simulink model "decoder_microinstruction_counter"  (R2020a)
settings: Solver=VariableStepAuto  StartTime=0.0  StopTime=inf  RelTol=1e-3
libraries: simulink_extras x1, dspswit3 x1, commutil2 x1
settings Model: EnablePacing=on  PacingRate=0.900000  Creator=F1  LastModifiedBy=F1

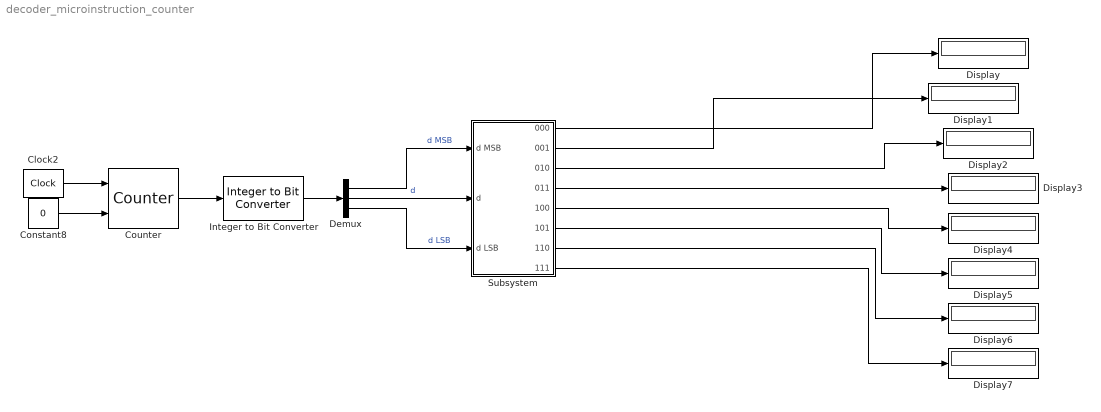
== system decoder_microinstruction_counter ==
  Clock2 : simulink_extras/Flip Flops/Clock  period=2
  Constant8 : Constant  Value=0
  Counter : dspswit3/Counter  Direction=Up  CountEvent=Rising edge  CounterSize=User defined  MaxCount=6  InitialCount=0  Output=Count  HitValue=32  ResetInput=on  SamplesPerFrame=1  Ts=1  CntDtype=int16  HitDtype=Logical
  Demux : Demux  Outputs=3
  Display{,1..7} (8 alike) : Display
  Integer to Bit Converter : commutil2/Integer to Bit Converter  nbits=3  signedInputValues=Unsigned  bitOrder=MSB first  outDtype=Inherit via internal rule
  Subsystem : Subsystem
  wires:
  Clock2/1 -> Counter/1
  Counter/1 -> Integer to Bit Converter/1
  Integer to Bit Converter/1 -> Demux/1
  Constant8/1 -> Counter/2
  Demux/1 -> Subsystem/1(d MSB)  "d MSB"
  Demux/2 -> Subsystem/2(d)  "d"
  Demux/3 -> Subsystem/3(d LSB)  "d LSB"
  Subsystem/1(000) -> Display/1
  Subsystem/2(001) -> Display1/1
  Subsystem/3(010) -> Display2/1
  Subsystem/4(011) -> Display3/1
  Subsystem/5(100) -> Display4/1
  Subsystem/6(101) -> Display5/1
  Subsystem/7(110) -> Display6/1
  Subsystem/8(111) -> Display7/1

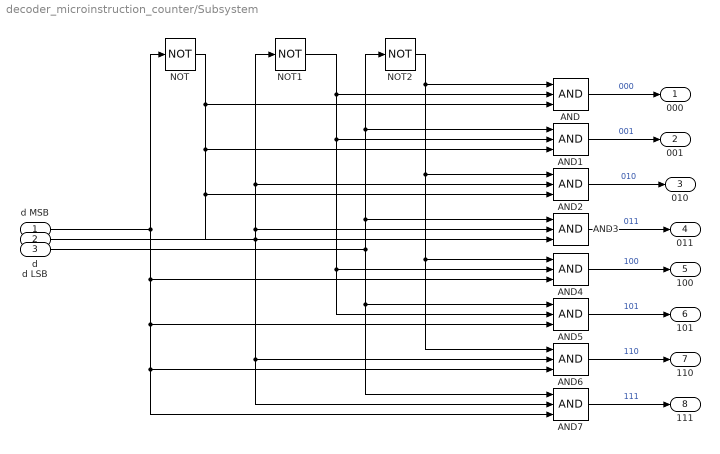
== system decoder_microinstruction_counter/Subsystem ==
  d MSB : Inport
  d : Inport  Port=2
  d LSB : Inport  Port=3
  AND{,1..7} (8 alike) : Logic  Inputs=3  IconShape=distinctive  AllPortsSameDT=off  OutDataTypeStr=boolean
  NOT : Logic  Operator=NOT  IconShape=distinctive  AllPortsSameDT=off  OutDataTypeStr=boolean
  NOT1 : Logic  Operator=NOT  IconShape=distinctive  AllPortsSameDT=off  OutDataTypeStr=boolean
  NOT2 : Logic  Operator=NOT  IconShape=distinctive  AllPortsSameDT=off  OutDataTypeStr=boolean
  000 : Outport
  001 : Outport  Port=2
  010 : Outport  Port=3
  011 : Outport  Port=4
  100 : Outport  Port=5
  101 : Outport  Port=6
  110 : Outport  Port=7
  111 : Outport  Port=8
  wires:
  d LSB/1 -> AND7/1, AND5/1, NOT2/1, AND1/1, AND3/1
  NOT/1 -> AND/3, AND1/3, AND3/3, AND2/3
  AND1/1 -> 001/1  "001"
  AND5/1 -> 101/1  "101"
  AND3/1 -> 011/1  "011"
  d/1 -> AND7/2, AND6/2, NOT1/1, AND2/2, AND3/2
  d MSB/1 -> AND7/3, AND6/3, AND5/3, AND4/3, NOT/1
  AND7/1 -> 111/1  "111"
  NOT1/1 -> AND5/2, AND4/2, AND1/2, AND/2
  AND4/1 -> 100/1  "100"
  NOT2/1 -> AND2/1, AND6/1, AND4/1, AND/1
  AND/1 -> 000/1  "000"
  AND2/1 -> 010/1  "010"
  AND6/1 -> 110/1  "110"
